simulink model "Model_New_PID"  (R2021b)
settings: Solver=VariableStepAuto  StartTime=0.0  StopTime=100  RelTol=1e-3
undefined symbols (not defined in the file): c, d, g, J, l, m, Rs
libraries: simulink x2, slpidlib x1
settings Model: Creator=Marcin  LastModifiedBy=Marcin

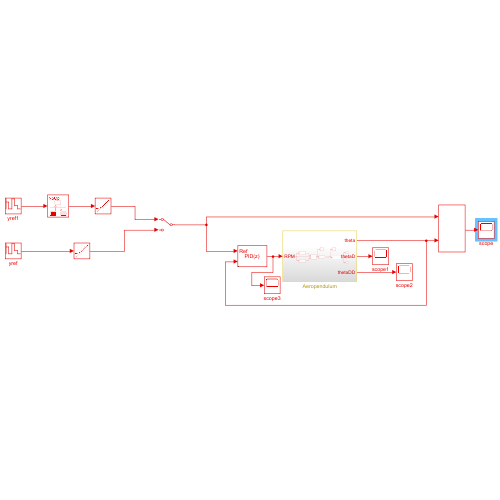
[thumbnail: Simulink's stored preview of the top-level diagram]
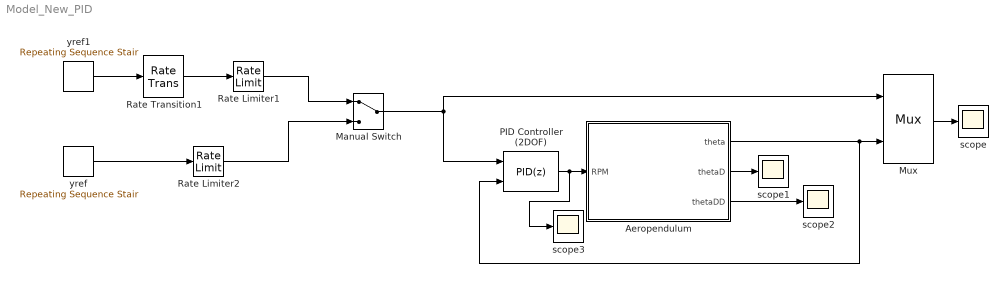
== system Model_New_PID ==
  Aeropendulum : Subsystem
  Manual Switch : ManualSwitch
  Mux : Mux  Inputs=2
  PID Controller (2DOF) : slpidlib/PID Controller (2DOF)  Controller=PID  Form=Parallel  TimeDomain=Discrete-time  UseExternalTs=off  SampleTime=-1  IntegratorMethod=Forward Euler  FilterMethod=Forward Euler  ControllerParametersSource=internal  P=5  I=26  D=0  UseFilter=on  N=100  b=1  c=1  TunerSelectOption=Transfer Function Based (PID Tuner App)  InitialConditionSource=internal  InitialConditionForIntegrator=0  InitialConditionForFilter=0  DifferentiatorICPrevScaledInput=0  ExternalReset=none  TrackingMode=off  Kt=1  LimitOutput=off  SatLimitsSource=internal  UpperSaturationLimit=inf  LowerSaturationLimit=-inf  LinearizeAsGain=on  AntiWindupMode=none  Kb=1  POutMin=[]  POutMax=[]  IOutMin=[]  IOutMax=[]  DOutMin=[]  DOutMax=[]  NOutMin=[]  NOutMax=[]  bOutMin=[]  bOutMax=[]  cOutMin=[]  cOutMax=[]  SumOutMin=[]  SumOutMax=[]  SaturationOutMin=[]  SaturationOutMax=[]  PParamMin=[]  PParamMax=[]  IParamMin=[]  IParamMax=[]  DParamMin=[]  DParamMax=[]  NParamMin=[]  NParamMax=[]  bParamMin=[]  bParamMax=[]  cParamMin=[]  cParamMax=[]  KbParamMin=[]  KbParamMax=[]  KtParamMin=[]  KtParamMax=[]  KbOutMin=[]  KbOutMax=[]  KtOutMin=[]  KtOutMax=[]  IntegratorOutMin=[]  IntegratorOutMax=[]  FilterOutMin=[]  FilterOutMax=[]  SumI1OutMin=[]  SumI1OutMax=[]  SumI2OutMin=[]  SumI2OutMax=[]  SumI3OutMin=[]  SumI3OutMax=[]  SumI4OutMin=[]  SumI4OutMax=[]  SumDOutMin=[]  SumDOutMax=[]  Sum1OutMin=[]  Sum1OutMax=[]  Sum2OutMin=[]  Sum2OutMax=[]  Sum3OutMin=[]  Sum3OutMax=[]  DifferentiatorOutMin=[]  DifferentiatorOutMax=[]  FilterDiffOutCoefMin=[]  FilterDiffOutCoefMax=[]  ReciprocalOutMin=[]  ReciprocalOutMax=[]  SumDenOutMin=[]  SumDenOutMax=[]  SumNumOutMin=[]  SumNumOutMax=[]  DivideOutMin=[]  DivideOutMax=[]  UdiffTsProdOutMin=[]  UdiffTsProdOutMax=[]  NTsProdOutMin=[]  NTsProdOutMax=[]  UintegralTsProdOutMin=[]  UintegralTsProdOutMax=[]  UngainTsProdOutMin=[]  UngainTsProdOutMax=[]  IntegratorContinuousStateAttributes=''  IntegratorStateMustResolveToSignalObject=off  IntegratorRTWStateStorageClass=Auto  FilterContinuousStateAttributes=''  FilterStateMustResolveToSignalObject=off  FilterRTWStateStorageClass=Auto  ParallelPVariant=InternalParameters  IdealPVariant=Disabled  IVariant=InternalParameters  DVariant=InternalParameters  bVariant=InternalParameters  cVariant=InternalParameters  IntegratorVariant=Discrete  SatVariant=Disabled  AWVariant=Passthrough  PCopyVariant=Disabled  TRVariant=Disabled  FdbkBlocksVariant=Forward  IdealPFdbkVariant=Disabled  SatFdbkVariant=Disabled  DerivativeFilterVariant=ForwardEulerFilter  NVariant=InternalParameters  NCopyVariant=Disabled  FilterICVariant=InternalICsFilter  IntegratorICVariant=InternalICs  ExternalResetVariant=Disabled  TRSumVariant=Passthrough  SumFdbkVariant=Disabled  SumVariant=Sum_PID  TsampFilterVariant=InternalTs  TsampNgainVariant=Passthrough  TsampIntegralVariant=Passthrough  ExternalSaturationOutDataTypeStr=Inherit: Same as second input
      settings: SourceProductBaseCode=SL
  Rate Limiter1 : RateLimiter  RisingSlewLimit=Rs  FallingSlewLimit=-Rs  SampleTimeMode=inherited
  Rate Limiter2 : RateLimiter  RisingSlewLimit=5  FallingSlewLimit=-5  SampleTimeMode=inherited
  Rate Transition1 : RateTransition  InitialCondition=10  OutPortSampleTime=Ts
  scope{,1..3} (4 alike) : Scope
  yref : simulink/Sources/Repeating Sequence Stair  OutValues=input_yref_vector  tsamp=Ts  OutMin=[]  OutMax=[]  OutDataTypeStr=double  OutputDataTypeScalingMode=double  OutDataType=fixdt(0,8)  ConRadixGroup=Best Precision: Vector-wise  OutScaling=2^-12
  yref1 : simulink/Sources/Repeating Sequence Stair  OutValues=input_yref_vector  tsamp=Ts  OutMin=[]  OutMax=[]  OutDataTypeStr=double  OutputDataTypeScalingMode=double  OutDataType=fixdt(0,8)  ConRadixGroup=Best Precision: Vector-wise  OutScaling=2^-12
  wires:
  yref/1 -> Rate Limiter2/1
  PID Controller (2DOF)/1 -> scope3/1, Aeropendulum/1(RPM)
  Mux/1 -> scope/1
  Aeropendulum/1(theta) -> PID Controller (2DOF)/2, Mux/2
  Aeropendulum/2(thetaD) -> scope1/1
  Aeropendulum/3(thetaDD) -> scope2/1
  yref1/1 -> Rate Transition1/1
  Rate Transition1/1 -> Rate Limiter1/1
  Rate Limiter1/1 -> Manual Switch/1
  Rate Limiter2/1 -> Manual Switch/2
  Manual Switch/1 -> Mux/1, PID Controller (2DOF)/1

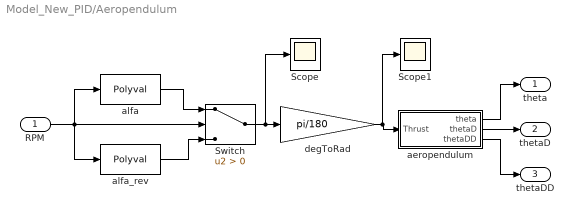
== system Model_New_PID/Aeropendulum ==
  RPM : Inport
  Scope : Scope
  Scope1 : Scope
  Switch : Switch  Criteria=u2 > Threshold
  aeropendulum : Subsystem
  alfa : Polyval  Coefs="[3.04986021927422e-06,  -0.00476887717971010 , 2.51670431281220]"
  alfa_rev : Polyval  Coefs="[-5.46944010985214e-06,\t-0.00938361577873603,\t-2.43262552689868]"
  degToRad : Gain  Gain=pi/180
  theta : Outport
  thetaD : Outport  Port=2
  thetaDD : Outport  Port=3
  wires:
  alfa/1 -> Switch/1
  RPM/1 -> alfa_rev/1, alfa/1, Switch/2
  Switch/1 -> Scope/1, degToRad/1
  degToRad/1 -> Scope1/1, aeropendulum/1(Thrust)
  alfa_rev/1 -> Switch/3
  aeropendulum/1(theta) -> theta/1
  aeropendulum/2(thetaD) -> thetaD/1
  aeropendulum/3(thetaDD) -> thetaDD/1

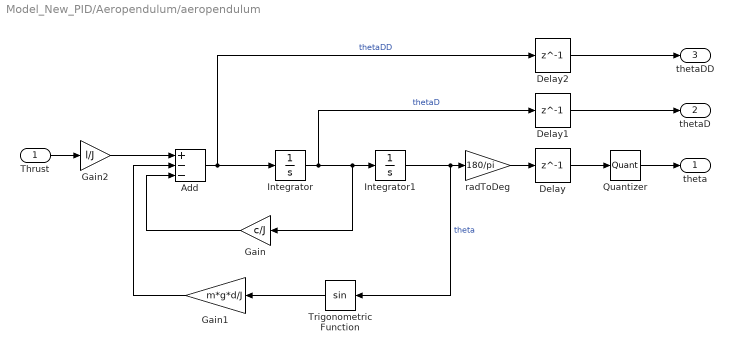
== system Model_New_PID/Aeropendulum/aeropendulum ==
  Thrust : Inport
  Add : Sum  Inputs=+--
  Delay : Delay  DelayLength=1  InitialCondition=0
  Delay1 : Delay  DelayLength=1  InitialCondition=0
  Delay2 : Delay  DelayLength=1  InitialCondition=0
  Gain : Gain  Gain=c/J
  Gain1 : Gain  Gain=m*g*d/J
  Gain2 : Gain  Gain=l/J
  Integrator : Integrator
  Integrator1 : Integrator
  Quantizer : Quantizer  QuantizationInterval=0.08791209
  Trigonometric Function : Trigonometry
  radToDeg : Gain  Gain=180/pi
  theta : Outport
  thetaD : Outport  Port=2
  thetaDD : Outport  Port=3
  wires:
  Thrust/1 -> Gain2/1
  Integrator/1 -> Delay1/1, Gain/1, Integrator1/1  "thetaD"
  Integrator1/1 -> Trigonometric Function/1, radToDeg/1  "theta"
  Add/1 -> Delay2/1, Integrator/1  "thetaDD"
  Gain1/1 -> Add/2
  Trigonometric Function/1 -> Gain1/1
  Gain/1 -> Add/3
  Gain2/1 -> Add/1
  radToDeg/1 -> Delay/1
  Delay1/1 -> thetaD/1
  Delay2/1 -> thetaDD/1
  Delay/1 -> Quantizer/1
  Quantizer/1 -> theta/1
